simulink model "Light_Buoy_test"  (Simulink 7.3)
settings: Solver=FixedStepDiscrete  StartTime=0.0  StopTime=inf  MaxStep=0.2  RelTol=1e-3
undefined symbols (not defined in the file): strel
libraries: dspmtrx3 x2, simulink x2, vipmorphops x1, vipstatistics x1, dspstat3 x1
settings Model: Creator=gclayton  LastModifiedBy=wildcat
settings DebuggingCC: InheritedTsInSrcMsg=none
settings RTWCC: SystemTargetFile=rlnx.tlc  GenCodeOnly=on  TemplateMakefile=rlnx_ubuntu.tmf  Description=Linux Real-Time Target  ProcessScript=rlnx_make_rtw_hook
settings RTWCC: CustomInclude=|
  | /usr/local/include/opencv/
  | /usr/local/include/
settings CodeAppCC: GenerateComments=off  SimulinkBlockComments=off
settings STFCustomTargetCC: ModelReferenceCompliant=off  MatFileLogging=on  SystemTargetFile=rlnx.tlc
settings GRTTargetCC: ModelReferenceCompliant=off  ParMdlRefBuildCompliant=off  CompOptLevelCompliant=off
settings CustomProperty: DataType=string  Value=-lm -ldl /usr/local/lib/libopencv_highgui.so.2.4 /usr/local/lib/libopencv_core.so.2.4 /usr/local/lib/libopencv_imgproc.so.2.4
settings EnumStrPairs: String=PC

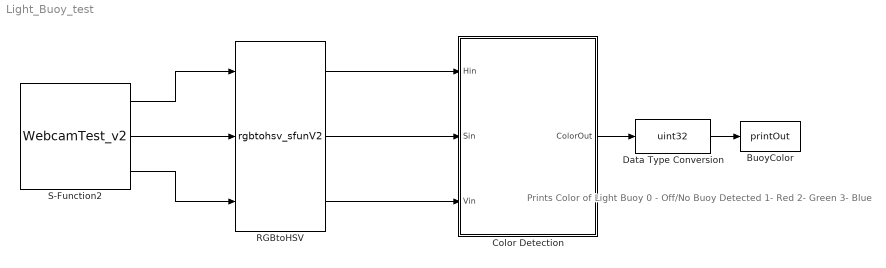
== system Light_Buoy_test ==
  note: Prints Color of Light Buoy
      | 0 - Off/No Buoy Detected
      | 1- Red
      | 2- Green
      | 3- Blue
  BuoyColor : S-Function  FunctionName=printOut  EnableBusSupport=off
  Color Detection : Subsystem
  Data Type Conversion : DataTypeConversion  OutDataTypeMode=uint32  OutDataType=fixdt(1, 16)  OutScaling=2^0  OutDataTypeStr=uint32
  RGBtoHSV : S-Function  FunctionName=rgbtohsv_sfunV2  EnableBusSupport=off
  S-Function2 : S-Function  FunctionName=WebcamTest_v2  EnableBusSupport=off
  wires:
  RGBtoHSV/2 -> Color Detection/2(Sin)
  RGBtoHSV/3 -> Color Detection/3(Vin)
  RGBtoHSV/1 -> Color Detection/1(Hin)
  S-Function2/3 -> RGBtoHSV/3
  S-Function2/2 -> RGBtoHSV/2
  S-Function2/1 -> RGBtoHSV/1
  Color Detection/1(ColorOut) -> Data Type Conversion/1
  Data Type Conversion/1 -> BuoyColor/1

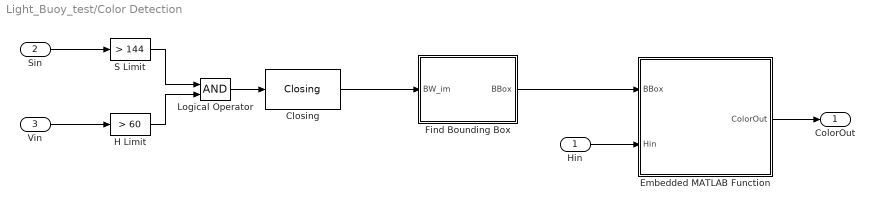
== system Light_Buoy_test/Color Detection ==
  Hin : Inport  OutDataType=fixdt(1, 16)  OutScaling=2^0
  Sin : Inport  Port=2  OutDataType=fixdt(1, 16)  OutScaling=2^0
  Vin : Inport  Port=3  OutDataType=fixdt(1, 16)  OutScaling=2^0
  Closing : vipmorphops/Closing  nhoodsrc=Specify via dialog  strel=strel('square',12)
  Embedded MATLAB Function : Stateflow chart
  Find Bounding Box : Subsystem
  H Limit : simulink/Logic and Bit Operations/Compare To Constant  SystemSampleTime=-1  relop=>  const=60  LogicOutDataTypeMode=uint8  ZeroCross=off
  Logical Operator : Logic  AllPortsSameDT=off  OutDataTypeMode=boolean  LogicDataType=fixdt(0, 8)  OutDataTypeStr=boolean
  S Limit : simulink/Logic and Bit Operations/Compare To Constant  SystemSampleTime=-1  relop=>  const=144  LogicOutDataTypeMode=uint8  ZeroCross=off
  ColorOut : Outport  OutDataType=fixdt(1, 16)  OutScaling=2^0
  wires:
  Sin/1 -> S Limit/1
  Vin/1 -> H Limit/1
  S Limit/1 -> Logical Operator/1
  H Limit/1 -> Logical Operator/2
  Logical Operator/1 -> Closing/1
  Closing/1 -> Find Bounding Box/1(BW_im)
  Find Bounding Box/1(BBox) -> Embedded MATLAB Function/1(BBox)
  Hin/1 -> Embedded MATLAB Function/2(Hin)
  Embedded MATLAB Function/1(ColorOut) -> ColorOut/1

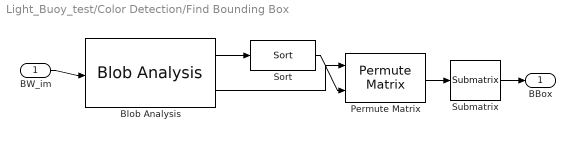
== system Light_Buoy_test/Color Detection/Find Bounding Box ==
  BW_im : Inport
  Blob Analysis : vipstatistics/Blob Analysis  DialogController=vipDDGCreate  DialogControllerArgs=DataTag0  area=on  centroid=off  bBox=on  majorAxis=off  minorAxis=off  angle=off  eccentricity=off  equivDiameterSq=off  extent=off  perimeter=off  maxBlobs=4  warnIfNumBlobsExceeded=on  isCount=off  useMinArea=on  minArea=30  useMaxArea=off  maxArea=intmax('uint32')  excludeBorderBlob=off  outDT=double  isOutVarDim=off  isFill=on  fillValues=-1  conn=8  isLabel=off  outputMode=Binary point scaling  outputWordLength=32  outputFracLength=16  firstCoeffMode=Binary point scaling  firstCoeffWordLength=16  firstCoeffFracLength=14  secondCoeffMode=Binary point scaling  secondCoeffWordLength=32  secondCoeffFracLength=16  accumMode=Binary point scaling  accumWordLength=32  accumFracLength=0  prodOutputMode=Binary point scaling  prodOutputWordLength=32  prodOutputFracLength=16  roundingMode=Floor  overflowMode=off
  Permute Matrix : dspmtrx3/Permute Matrix  mode=Columns  ZeroOneIdxMode=One-based  errmode=Clip index  checkDims=off
  Sort : dspstat3/Sort  DialogController=dspDDGCreate  DialogControllerArgs=DataTag1  otype=Index  dir=Descending  sortAlg=Quick sort  roundingMode=Floor  overflowMode=off
  Submatrix : dspmtrx3/Submatrix  RowSpan=All rows  RowStartMode=First  RowStartIndex=1  RowEndMode=Last  RowEndIndex=1  ColSpan=One column  ColStartMode=First  ColStartIndex=1  ColEndMode=Last  ColEndIndex=1
  BBox : Outport
  wires:
  Blob Analysis/1 -> Sort/1
  Sort/1 -> Permute Matrix/2
  Blob Analysis/2 -> Permute Matrix/1
  Permute Matrix/1 -> Submatrix/1
  BW_im/1 -> Blob Analysis/1
  Submatrix/1 -> BBox/1

== matlab function Color Detection/Embedded MATLAB Function ==
  data: BBox input double; Hin input double; ColorOut output double
function ColorOut = ColorA(BBox,Hin)
% Determine color 

% Used to generate image to check if correct
% RMask = zeros(480,640);
% GMask = zeros(480,640);
% BMask = zeros(480,640);

% Obtain upper left row and column, 
% and height and width of Bounding Box
row = BBox(1);
column = BBox(2);
height = BBox(3);
width = BBox(4);

R_Count = 0;
G_Count = 0;
B_Count = 0;
ColorOut = 0;

% Check for color within Bounding Box
for i = row:(row+height)
    for j = column:(column+width)
        
        % Create Red Image
        if (Hin(i,j) >= 250 || Hin(i,j) < 4)
            %RMask(i,j) = 1;
            R_Count = R_Count+1;
        end
        
        % Create Green Image
        if (Hin(i,j) > 75 && Hin(i,j) < 95)
            %GMask(i,j) = 1;
            G_Count = G_Count+1;
        end
        
        % Create Blue Image
        if (Hin(i,j) > 160 && Hin(i,j) < 175)
            %BMask(i,j) = 1;
            B_Count = B_Count+1;
        end
        
    end
end

if (R_Count > 30)
    ColorOut = 1;
elseif (G_Count > 30)
    ColorOut = 2;
elseif (B_Count > 30)
    ColorOut = 3;
else
    ColorOut = 0;
end
